simulink model "Casc_Filter_x4"  (Simulink 6.6)
settings: Solver=ode45  StartTime=0.0  StopTime=4100/sampling_freq  RelTol=1e-3
values from neighbouring files (symbols this model uses):
  filter_clk = sampling_freq*clk_mult    (= 144000000)    [Casecade_Taps.m]
  h_g = round(h_g*2^17)/2^17    [Casecade_Taps.m]
  h_k = round(h_k*2^17)/2^17    [Casecade_Taps.m]
  sampling_freq = 48e6    (= 48000000)    [Casecade_Taps.m]
undefined symbols (not defined in the file or in its folder): A, B, Fs, get, PCIN
libraries: xbsIndex_r4 x839, dspsnks4 x5, dspsrcs4 x1, simulink x1
(part 2 of 8)

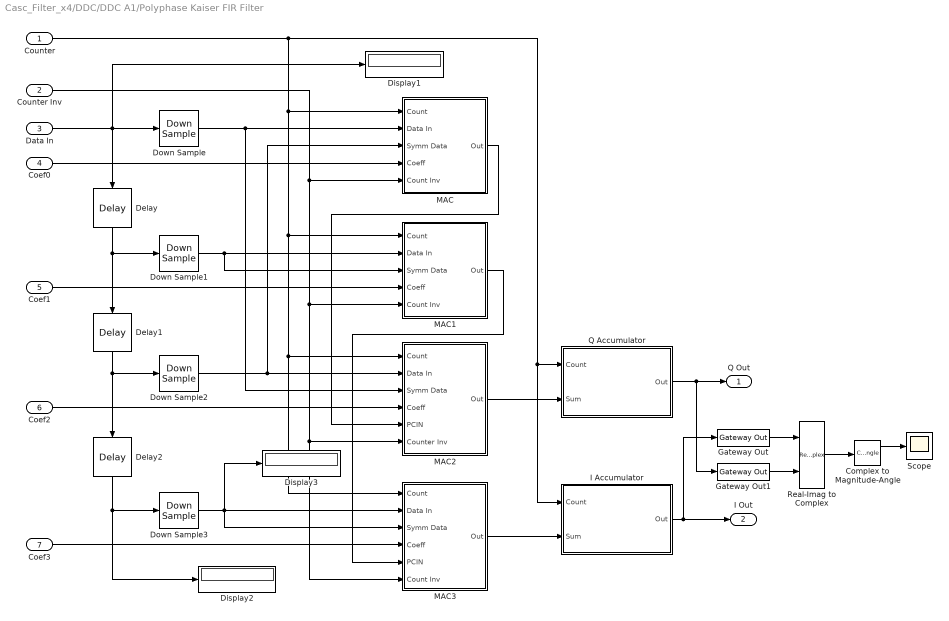
== system Casc_Filter_x4/DDC/DDC A1/Polyphase Kaiser FIR Filter ==
  Counter : Inport
  Counter Inv : Inport  Port=2
  Data In : Inport  Port=3
  Coef0 : Inport  Port=4
  Coef1 : Inport  Port=5
  Coef2 : Inport  Port=6
  Coef3 : Inport  Port=7
  Complex to Magnitude-Angle : ComplexToMagnitudeAngle
  Delay : xbsIndex_r4/Delay  Orientation=down  en=off  latency=1  dbl_ovrd=off  reg_retiming=off  block_type=delay
      settings: infoedit=Hardware notes: A delay line is a chain, each link of which is an SRL16 followed by a flip-flop. If register retiming is enabled, the delay line is a chain of flip-flops.  block_version=8.2
  Delay1 : xbsIndex_r4/Delay  Orientation=down  en=off  latency=1  dbl_ovrd=off  reg_retiming=off  block_type=delay
      settings: infoedit=Hardware notes: A delay line is a chain, each link of which is an SRL16 followed by a flip-flop. If register retiming is enabled, the delay line is a chain of flip-flops.  block_version=8.2
  Delay2 : xbsIndex_r4/Delay  Orientation=down  en=off  latency=1  dbl_ovrd=off  reg_retiming=off  block_type=delay
      settings: infoedit=Hardware notes: A delay line is a chain, each link of which is an SRL16 followed by a flip-flop. If register retiming is enabled, the delay line is a chain of flip-flops.  block_version=8.2
  Display1 : Display
  Display2 : Display
  Display3 : Display
  Down Sample{,1..3} (4 alike) : xbsIndex_r4/Down Sample  sample_ratio=4  sample_phase="Last Value of Frame  (most efficient)"  en=off  latency=1  dbl_ovrd=off  block_type=dsamp
      settings: block_version=8.2
  Gateway Out : xbsIndex_r4/Gateway Out  hdl_port=off  timing_constraint=None  locs_specified=off  LOCs={}  block_type=gatewayout
      settings: infoedit="Gateway out block.  Converts Xilinx fixed point inputs into ouputs of type Simulink integer, double, or fixed point.<P><P>Hardware notes:  In hardware these blocks become top level output ports or are discarded, depending on how they are configured."  block_version=8.2
  Gateway Out1 : xbsIndex_r4/Gateway Out  hdl_port=off  timing_constraint=None  locs_specified=off  LOCs={}  block_type=gatewayout
      settings: infoedit="Gateway out block.  Converts Xilinx fixed point inputs into ouputs of type Simulink integer, double, or fixed point.<P><P>Hardware notes:  In hardware these blocks become top level output ports or are discarded, depending on how they are configured."  block_version=8.2
  I Accumulator : Subsystem
  MAC : Subsystem
  MAC1 : Subsystem
  MAC2 : Subsystem
  MAC3 : Subsystem
  Q Accumulator : Subsystem
  Real-Imag to Complex : RealImagToComplex
  Scope : Scope
  Q Out : Outport
  I Out : Outport  Port=2
  wires:
  Data In/1 -> Down Sample/1, Delay/1, Display1/1
  Delay/1 -> Down Sample1/1, Delay1/1
  Delay1/1 -> Down Sample2/1, Delay2/1
  Delay2/1 -> Down Sample3/1, Display2/1
  Coef0/1 -> MAC/4(Coeff)
  Coef1/1 -> MAC1/4(Coeff)
  I Accumulator/1(Out) -> I Out/1, Gateway Out/1
  Counter/1 -> MAC3/1(Count), MAC2/1(Count), MAC1/1(Count), MAC/1(Count), Q Accumulator/1(Count), I Accumulator/1(Count)
  Coef2/1 -> MAC2/4(Coeff)
  Coef3/1 -> MAC3/4(Coeff)
  Q Accumulator/1(Out) -> Q Out/1, Gateway Out1/1
  Down Sample/1 -> MAC/2(Data In), MAC2/3(Symm Data)
  Down Sample1/1 -> MAC1/3(Symm Data), MAC1/2(Data In)
  Down Sample2/1 -> MAC/3(Symm Data), MAC2/2(Data In)
  Down Sample3/1 -> MAC3/3(Symm Data), MAC3/2(Data In), Display3/1
  MAC/1(Out) -> MAC2/5(PCIN)
  MAC2/1(Out) -> Q Accumulator/2(Sum)
  MAC1/1(Out) -> MAC3/5(PCIN)
  MAC3/1(Out) -> I Accumulator/2(Sum)
  Counter Inv/1 -> MAC/5(Count Inv), MAC1/5(Count Inv), MAC2/6(Counter Inv), MAC3/6(Count Inv)
  Real-Imag to Complex/1 -> Complex to Magnitude-Angle/1
  Complex to Magnitude-Angle/1 -> Scope/1
  Gateway Out/1 -> Real-Imag to Complex/1
  Gateway Out1/1 -> Real-Imag to Complex/2

== system Casc_Filter_x4/DDC/DDC B/Gaussian FIR Filters ==
  Counter : Inport
  Counter Inv : Inport  Port=2
  Q In : Inport  Port=3
  Coef0 : Inport  Port=4
  Coef1 : Inport  Port=5
  Coef2 : Inport  Port=6
  I In : Inport  Port=7
  Gaussian FIR Filter : Subsystem
  Gaussian FIR Filter1 : Subsystem
  I Out : Outport
  Q Out : Outport  Port=2
  wires:
  Counter/1 -> Gaussian FIR Filter/1(Counter), Gaussian FIR Filter1/1(Counter)
  Counter Inv/1 -> Gaussian FIR Filter/2(Counter Inv), Gaussian FIR Filter1/2(Counter Inv)
  Q In/1 -> Gaussian FIR Filter/3(Data In)
  I In/1 -> Gaussian FIR Filter1/3(Data In)
  Gaussian FIR Filter/1(Data Out) -> Q Out/1
  Gaussian FIR Filter1/1(Data Out) -> I Out/1
  Coef0/1 -> Gaussian FIR Filter/4(Coef0), Gaussian FIR Filter1/4(Coef0)
  Coef1/1 -> Gaussian FIR Filter/5(Coef1), Gaussian FIR Filter1/5(Coef1)
  Coef2/1 -> Gaussian FIR Filter/6(Coef2), Gaussian FIR Filter1/6(Coef2)

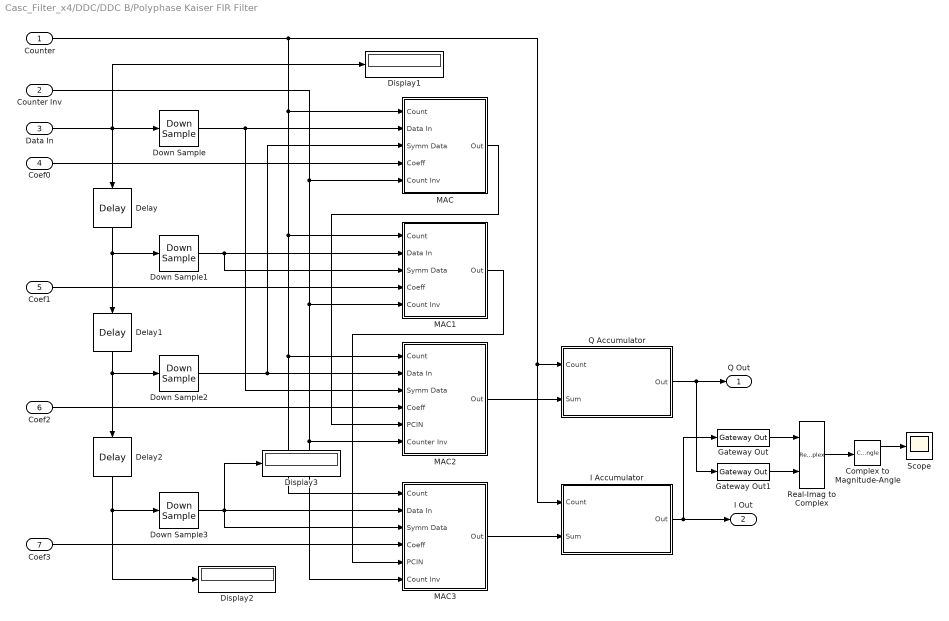
== system Casc_Filter_x4/DDC/DDC B/Polyphase Kaiser FIR Filter ==
  Counter : Inport
  Counter Inv : Inport  Port=2
  Data In : Inport  Port=3
  Coef0 : Inport  Port=4
  Coef1 : Inport  Port=5
  Coef2 : Inport  Port=6
  Coef3 : Inport  Port=7
  Complex to Magnitude-Angle : ComplexToMagnitudeAngle
  Delay : xbsIndex_r4/Delay  Orientation=down  en=off  latency=1  dbl_ovrd=off  reg_retiming=off  block_type=delay
      settings: infoedit=Hardware notes: A delay line is a chain, each link of which is an SRL16 followed by a flip-flop. If register retiming is enabled, the delay line is a chain of flip-flops.  block_version=8.2
  Delay1 : xbsIndex_r4/Delay  Orientation=down  en=off  latency=1  dbl_ovrd=off  reg_retiming=off  block_type=delay
      settings: infoedit=Hardware notes: A delay line is a chain, each link of which is an SRL16 followed by a flip-flop. If register retiming is enabled, the delay line is a chain of flip-flops.  block_version=8.2
  Delay2 : xbsIndex_r4/Delay  Orientation=down  en=off  latency=1  dbl_ovrd=off  reg_retiming=off  block_type=delay
      settings: infoedit=Hardware notes: A delay line is a chain, each link of which is an SRL16 followed by a flip-flop. If register retiming is enabled, the delay line is a chain of flip-flops.  block_version=8.2
  Display1 : Display
  Display2 : Display
  Display3 : Display
  Down Sample{,1..3} (4 alike) : xbsIndex_r4/Down Sample  sample_ratio=4  sample_phase="Last Value of Frame  (most efficient)"  en=off  latency=1  dbl_ovrd=off  block_type=dsamp
      settings: block_version=8.2
  Gateway Out : xbsIndex_r4/Gateway Out  hdl_port=off  timing_constraint=None  locs_specified=off  LOCs={}  block_type=gatewayout
      settings: infoedit="Gateway out block.  Converts Xilinx fixed point inputs into ouputs of type Simulink integer, double, or fixed point.<P><P>Hardware notes:  In hardware these blocks become top level output ports or are discarded, depending on how they are configured."  block_version=8.2
  Gateway Out1 : xbsIndex_r4/Gateway Out  hdl_port=off  timing_constraint=None  locs_specified=off  LOCs={}  block_type=gatewayout
      settings: infoedit="Gateway out block.  Converts Xilinx fixed point inputs into ouputs of type Simulink integer, double, or fixed point.<P><P>Hardware notes:  In hardware these blocks become top level output ports or are discarded, depending on how they are configured."  block_version=8.2
  I Accumulator : Subsystem
  MAC : Subsystem
  MAC1 : Subsystem
  MAC2 : Subsystem
  MAC3 : Subsystem
  Q Accumulator : Subsystem
  Real-Imag to Complex : RealImagToComplex
  Scope : Scope
  Q Out : Outport
  I Out : Outport  Port=2
  wires:
  Data In/1 -> Down Sample/1, Delay/1, Display1/1
  Delay/1 -> Down Sample1/1, Delay1/1
  Delay1/1 -> Down Sample2/1, Delay2/1
  Delay2/1 -> Down Sample3/1, Display2/1
  Coef0/1 -> MAC/4(Coeff)
  Coef1/1 -> MAC1/4(Coeff)
  I Accumulator/1(Out) -> I Out/1, Gateway Out/1
  Counter/1 -> MAC3/1(Count), MAC2/1(Count), MAC1/1(Count), MAC/1(Count), Q Accumulator/1(Count), I Accumulator/1(Count)
  Coef2/1 -> MAC2/4(Coeff)
  Coef3/1 -> MAC3/4(Coeff)
  Q Accumulator/1(Out) -> Q Out/1, Gateway Out1/1
  Down Sample/1 -> MAC/2(Data In), MAC2/3(Symm Data)
  Down Sample1/1 -> MAC1/3(Symm Data), MAC1/2(Data In)
  Down Sample2/1 -> MAC/3(Symm Data), MAC2/2(Data In)
  Down Sample3/1 -> MAC3/3(Symm Data), MAC3/2(Data In), Display3/1
  MAC/1(Out) -> MAC2/5(PCIN)
  MAC2/1(Out) -> Q Accumulator/2(Sum)
  MAC1/1(Out) -> MAC3/5(PCIN)
  MAC3/1(Out) -> I Accumulator/2(Sum)
  Counter Inv/1 -> MAC/5(Count Inv), MAC1/5(Count Inv), MAC2/6(Counter Inv), MAC3/6(Count Inv)
  Real-Imag to Complex/1 -> Complex to Magnitude-Angle/1
  Complex to Magnitude-Angle/1 -> Scope/1
  Gateway Out/1 -> Real-Imag to Complex/1
  Gateway Out1/1 -> Real-Imag to Complex/2

== system Casc_Filter_x4/DDC/DDC C/Gaussian FIR Filters ==
  Counter : Inport
  Counter Inv : Inport  Port=2
  Q In : Inport  Port=3
  Coef0 : Inport  Port=4
  Coef1 : Inport  Port=5
  Coef2 : Inport  Port=6
  I In : Inport  Port=7
  Gaussian FIR Filter : Subsystem
  Gaussian FIR Filter1 : Subsystem
  I Out : Outport
  Q Out : Outport  Port=2
  wires:
  Counter/1 -> Gaussian FIR Filter/1(Counter), Gaussian FIR Filter1/1(Counter)
  Counter Inv/1 -> Gaussian FIR Filter/2(Counter Inv), Gaussian FIR Filter1/2(Counter Inv)
  Q In/1 -> Gaussian FIR Filter/3(Data In)
  I In/1 -> Gaussian FIR Filter1/3(Data In)
  Gaussian FIR Filter/1(Data Out) -> Q Out/1
  Gaussian FIR Filter1/1(Data Out) -> I Out/1
  Coef0/1 -> Gaussian FIR Filter/4(Coef0), Gaussian FIR Filter1/4(Coef0)
  Coef1/1 -> Gaussian FIR Filter/5(Coef1), Gaussian FIR Filter1/5(Coef1)
  Coef2/1 -> Gaussian FIR Filter/6(Coef2), Gaussian FIR Filter1/6(Coef2)

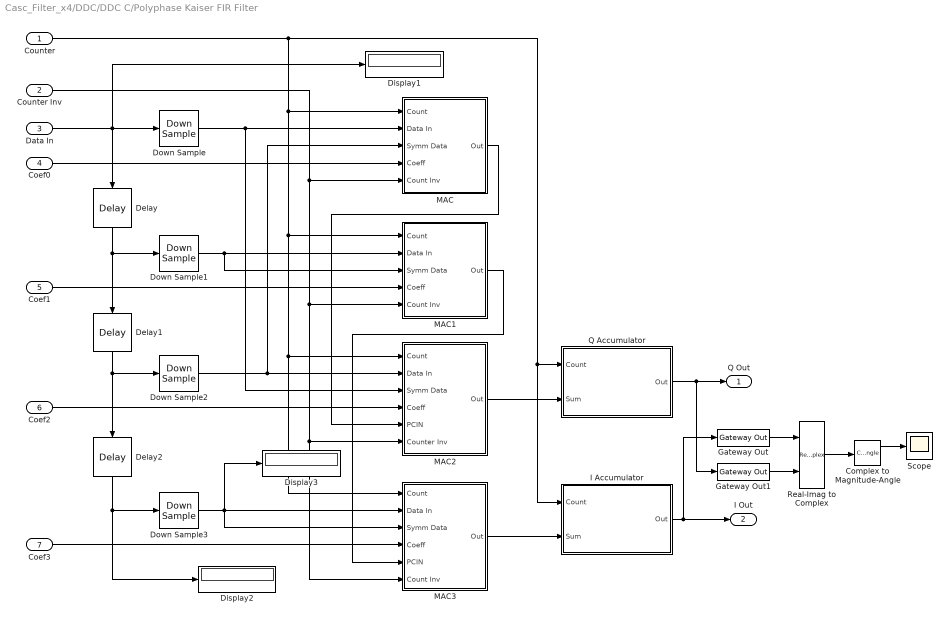
== system Casc_Filter_x4/DDC/DDC C/Polyphase Kaiser FIR Filter ==
  Counter : Inport
  Counter Inv : Inport  Port=2
  Data In : Inport  Port=3
  Coef0 : Inport  Port=4
  Coef1 : Inport  Port=5
  Coef2 : Inport  Port=6
  Coef3 : Inport  Port=7
  Complex to Magnitude-Angle : ComplexToMagnitudeAngle
  Delay : xbsIndex_r4/Delay  Orientation=down  en=off  latency=1  dbl_ovrd=off  reg_retiming=off  block_type=delay
      settings: infoedit=Hardware notes: A delay line is a chain, each link of which is an SRL16 followed by a flip-flop. If register retiming is enabled, the delay line is a chain of flip-flops.  block_version=8.2
  Delay1 : xbsIndex_r4/Delay  Orientation=down  en=off  latency=1  dbl_ovrd=off  reg_retiming=off  block_type=delay
      settings: infoedit=Hardware notes: A delay line is a chain, each link of which is an SRL16 followed by a flip-flop. If register retiming is enabled, the delay line is a chain of flip-flops.  block_version=8.2
  Delay2 : xbsIndex_r4/Delay  Orientation=down  en=off  latency=1  dbl_ovrd=off  reg_retiming=off  block_type=delay
      settings: infoedit=Hardware notes: A delay line is a chain, each link of which is an SRL16 followed by a flip-flop. If register retiming is enabled, the delay line is a chain of flip-flops.  block_version=8.2
  Display1 : Display
  Display2 : Display
  Display3 : Display
  Down Sample{,1..3} (4 alike) : xbsIndex_r4/Down Sample  sample_ratio=4  sample_phase="Last Value of Frame  (most efficient)"  en=off  latency=1  dbl_ovrd=off  block_type=dsamp
      settings: block_version=8.2
  Gateway Out : xbsIndex_r4/Gateway Out  hdl_port=off  timing_constraint=None  locs_specified=off  LOCs={}  block_type=gatewayout
      settings: infoedit="Gateway out block.  Converts Xilinx fixed point inputs into ouputs of type Simulink integer, double, or fixed point.<P><P>Hardware notes:  In hardware these blocks become top level output ports or are discarded, depending on how they are configured."  block_version=8.2
  Gateway Out1 : xbsIndex_r4/Gateway Out  hdl_port=off  timing_constraint=None  locs_specified=off  LOCs={}  block_type=gatewayout
      settings: infoedit="Gateway out block.  Converts Xilinx fixed point inputs into ouputs of type Simulink integer, double, or fixed point.<P><P>Hardware notes:  In hardware these blocks become top level output ports or are discarded, depending on how they are configured."  block_version=8.2
  I Accumulator : Subsystem
  MAC : Subsystem
  MAC1 : Subsystem
  MAC2 : Subsystem
  MAC3 : Subsystem
  Q Accumulator : Subsystem
  Real-Imag to Complex : RealImagToComplex
  Scope : Scope
  Q Out : Outport
  I Out : Outport  Port=2
  wires:
  Data In/1 -> Down Sample/1, Delay/1, Display1/1
  Delay/1 -> Down Sample1/1, Delay1/1
  Delay1/1 -> Down Sample2/1, Delay2/1
  Delay2/1 -> Down Sample3/1, Display2/1
  Coef0/1 -> MAC/4(Coeff)
  Coef1/1 -> MAC1/4(Coeff)
  I Accumulator/1(Out) -> I Out/1, Gateway Out/1
  Counter/1 -> MAC3/1(Count), MAC2/1(Count), MAC1/1(Count), MAC/1(Count), Q Accumulator/1(Count), I Accumulator/1(Count)
  Coef2/1 -> MAC2/4(Coeff)
  Coef3/1 -> MAC3/4(Coeff)
  Q Accumulator/1(Out) -> Q Out/1, Gateway Out1/1
  Down Sample/1 -> MAC/2(Data In), MAC2/3(Symm Data)
  Down Sample1/1 -> MAC1/3(Symm Data), MAC1/2(Data In)
  Down Sample2/1 -> MAC/3(Symm Data), MAC2/2(Data In)
  Down Sample3/1 -> MAC3/3(Symm Data), MAC3/2(Data In), Display3/1
  MAC/1(Out) -> MAC2/5(PCIN)
  MAC2/1(Out) -> Q Accumulator/2(Sum)
  MAC1/1(Out) -> MAC3/5(PCIN)
  MAC3/1(Out) -> I Accumulator/2(Sum)
  Counter Inv/1 -> MAC/5(Count Inv), MAC1/5(Count Inv), MAC2/6(Counter Inv), MAC3/6(Count Inv)
  Real-Imag to Complex/1 -> Complex to Magnitude-Angle/1
  Complex to Magnitude-Angle/1 -> Scope/1
  Gateway Out/1 -> Real-Imag to Complex/1
  Gateway Out1/1 -> Real-Imag to Complex/2

== system Casc_Filter_x4/DDC/Coefficients/Gaus Coef Mem/Select Decoder ==
  Run/Stop : Inport
  Wr/R : Inport  Port=2
  Sel : Inport  Port=3
  BitBasher : xbsIndex_r4/BitBasher  bitexpr=|  display_expr=off  sr_1=1  arith_type1=Unsigned  bin_pt1=0  sr_2=2  arith_type2=Unsigned  bin_pt2=0  sr_3=3  arith_type3=Unsigned  bin_pt3=0  sr_4=4  arith_type4=Unsigned  bin_pt4=0  dbl_ovrd=off  block_type=bitbasher
      | <html><head><meta name="qrichtext" content="1" /></head><body style="font-size:8pt;font-family:MS Shell Dlg">
      | <p>Sel0={Sel[0]}<br />Sel1={Sel[1]}<br /></p>
      | </body></html>
      settings: infoedit="Allows      extraction, concatenation and augmentation of bits"  block_version=VER_STRING_GOES_HERE
  Convert{,1..2,5} (4 alike) : xbsIndex_r4/Convert  arith_type=Boolean  n_bits=16  bin_pt=14  quantization=Truncate  overflow=Wrap  latency=0  dbl_ovrd=off  pipeline=off  block_type=convert
      settings: xl_area=[0 0 0 0 0 0 0]  block_version=VER_STRING_GOES_HERE
  Inverter : xbsIndex_r4/Inverter  en=off  latency=0  dbl_ovrd=off  block_type=inv
      settings: block_version=VER_STRING_GOES_HERE
  Inverter1 : xbsIndex_r4/Inverter  en=off  latency=0  dbl_ovrd=off  block_type=inv
      settings: block_version=VER_STRING_GOES_HERE
  Inverter2 : xbsIndex_r4/Inverter  en=off  latency=0  dbl_ovrd=off  block_type=inv
      settings: block_version=VER_STRING_GOES_HERE
  Logical : xbsIndex_r4/Logical  logical_function=AND  inputs=4  en=off  latency=0  precision=Full  arith_type=Unsigned  n_bits=16  bin_pt=0  align_bp=on  dbl_ovrd=off  block_type=logical
      settings: block_version=VER_STRING_GOES_HERE
  Logical1 : xbsIndex_r4/Logical  logical_function=AND  inputs=4  en=off  latency=0  precision=Full  arith_type=Unsigned  n_bits=16  bin_pt=0  align_bp=on  dbl_ovrd=off  block_type=logical
      settings: block_version=VER_STRING_GOES_HERE
  Logical2 : xbsIndex_r4/Logical  logical_function=AND  inputs=4  en=off  latency=0  precision=Full  arith_type=Unsigned  n_bits=16  bin_pt=0  align_bp=on  dbl_ovrd=off  block_type=logical
      settings: block_version=VER_STRING_GOES_HERE
  Logical3 : xbsIndex_r4/Logical  logical_function=AND  inputs=2  en=off  latency=0  precision=Full  arith_type=Unsigned  n_bits=16  bin_pt=0  align_bp=on  dbl_ovrd=off  block_type=logical
      settings: block_version=VER_STRING_GOES_HERE
  R_En : Outport
  Wr0 : Outport  Port=2
  Wr1 : Outport  Port=3
  Wr2 : Outport  Port=4
  wires:
  BitBasher/1 -> Convert/1
  BitBasher/2 -> Convert1/1
  Sel/1 -> BitBasher/1
  Logical/1 -> Wr0/1
  Logical1/1 -> Wr1/1
  Logical2/1 -> Wr2/1
  Wr/R/1 -> Convert2/1
  Convert/1 -> Inverter/1, Logical1/2
  Convert1/1 -> Inverter1/1, Logical2/3
  Convert2/1 -> Inverter2/1, Logical/1, Logical1/1, Logical2/1
  Inverter/1 -> Logical/2, Logical2/2
  Inverter1/1 -> Logical/3, Logical1/3
  Run/Stop/1 -> Convert5/1
  Convert5/1 -> Logical3/1, Logical/4, Logical1/4, Logical2/4
  Inverter2/1 -> Logical3/2
  Logical3/1 -> R_En/1

== system Casc_Filter_x4/DDC/Coefficients/Poly Coef Mem/Select Decoder ==
  Run/Stop : Inport
  Wr/R : Inport  Port=2
  Sel : Inport  Port=3
  BitBasher : xbsIndex_r4/BitBasher  bitexpr=|  display_expr=off  sr_1=1  arith_type1=Unsigned  bin_pt1=0  sr_2=2  arith_type2=Unsigned  bin_pt2=0  sr_3=3  arith_type3=Unsigned  bin_pt3=0  sr_4=4  arith_type4=Unsigned  bin_pt4=0  dbl_ovrd=off  block_type=bitbasher
      | <html><head><meta name="qrichtext" content="1" /></head><body style="font-size:8pt;font-family:MS Shell Dlg">
      | <p>Sel0={Sel[0]}<br />Sel1={Sel[1]}<br /></p>
      | </body></html>
      settings: infoedit="Allows      extraction, concatenation and augmentation of bits"  block_version=VER_STRING_GOES_HERE
  Convert{,1..2,4} (4 alike) : xbsIndex_r4/Convert  arith_type=Boolean  n_bits=16  bin_pt=14  quantization=Truncate  overflow=Wrap  latency=0  dbl_ovrd=off  pipeline=on  block_type=convert
      settings: xl_area=[0 0 0 0 0 0 0]  block_version=VER_STRING_GOES_HERE
  Inverter : xbsIndex_r4/Inverter  en=off  latency=0  dbl_ovrd=off  block_type=inv
      settings: block_version=VER_STRING_GOES_HERE
  Inverter1 : xbsIndex_r4/Inverter  en=off  latency=0  dbl_ovrd=off  block_type=inv
      settings: block_version=VER_STRING_GOES_HERE
  Inverter2 : xbsIndex_r4/Inverter  en=off  latency=0  dbl_ovrd=off  block_type=inv
      settings: block_version=VER_STRING_GOES_HERE
  Logical{,1..3} (4 alike) : xbsIndex_r4/Logical  logical_function=AND  inputs=4  en=off  latency=0  precision=Full  arith_type=Unsigned  n_bits=16  bin_pt=0  align_bp=on  dbl_ovrd=off  block_type=logical
      settings: block_version=VER_STRING_GOES_HERE
  Logical4 : xbsIndex_r4/Logical  logical_function=AND  inputs=2  en=off  latency=0  precision=Full  arith_type=Unsigned  n_bits=16  bin_pt=0  align_bp=on  dbl_ovrd=off  block_type=logical
      settings: block_version=VER_STRING_GOES_HERE
  R_En : Outport
  Wr0 : Outport  Port=2
  Wr1 : Outport  Port=3
  Wr2 : Outport  Port=4
  Wr3 : Outport  Port=5
  wires:
  BitBasher/1 -> Convert/1
  BitBasher/2 -> Convert1/1
  Sel/1 -> BitBasher/1
  Logical/1 -> Wr0/1
  Logical1/1 -> Wr1/1
  Logical2/1 -> Wr2/1
  Logical3/1 -> Wr3/1
  Wr/R/1 -> Convert2/1
  Convert/1 -> Inverter/1, Logical1/2, Logical3/2
  Convert1/1 -> Inverter1/1, Logical3/3, Logical2/3
  Convert2/1 -> Inverter2/1, Logical/1, Logical1/1, Logical2/1, Logical3/1
  Inverter/1 -> Logical/2, Logical2/2
  Inverter1/1 -> Logical/3, Logical1/3
  Run/Stop/1 -> Convert4/1
  Convert4/1 -> Logical4/1, Logical/4, Logical1/4, Logical2/4, Logical3/4
  Inverter2/1 -> Logical4/2
  Logical4/1 -> R_En/1

== system Casc_Filter_x4/DDC/DDC A/Gaussian FIR Filters/Gaussian FIR Filter ==
  Counter : Inport
  Counter Inv : Inport  Port=2
  Data In : Inport  Port=3
  Coef0 : Inport  Port=4
  Coef1 : Inport  Port=5
  Coef2 : Inport  Port=6
  Gaussian Accumulate : Subsystem
  Gaussian Mult : Subsystem
  Symmetric Data Flow : Subsystem
  Data Out : Outport
  wires:
  Counter/1 -> Gaussian Accumulate/1(Counter), Symmetric Data Flow/2(Counter)
  Gaussian Mult/1(Sum Out) -> Gaussian Accumulate/2(Data In)
  Symmetric Data Flow/1(Data 1) -> Gaussian Mult/1(Data 1)
  Symmetric Data Flow/2(Data 2) -> Gaussian Mult/2(Data 2)
  Data In/1 -> Symmetric Data Flow/1(Data In)
  Gaussian Accumulate/1(Data Out) -> Data Out/1
  Symmetric Data Flow/3(Data 3) -> Gaussian Mult/3(Data 3)
  Coef0/1 -> Gaussian Mult/4(Coeff 1)
  Coef1/1 -> Gaussian Mult/5(Coeff 2)
  Counter Inv/1 -> Symmetric Data Flow/3(Counter Inv)
  Coef2/1 -> Gaussian Mult/6(Coeff 3)

== system Casc_Filter_x4/DDC/DDC A/Gaussian FIR Filters/Gaussian FIR Filter1 ==
  Counter : Inport
  Counter Inv : Inport  Port=2
  Data In : Inport  Port=3
  Coef0 : Inport  Port=4
  Coef1 : Inport  Port=5
  Coef2 : Inport  Port=6
  Gaussian Accumulate : Subsystem
  Gaussian Mult : Subsystem
  Symmetric Data Flow : Subsystem
  Data Out : Outport
  wires:
  Counter/1 -> Gaussian Accumulate/1(Counter), Symmetric Data Flow/2(Counter)
  Gaussian Mult/1(Sum Out) -> Gaussian Accumulate/2(Data In)
  Symmetric Data Flow/1(Data 1) -> Gaussian Mult/1(Data 1)
  Symmetric Data Flow/2(Data 2) -> Gaussian Mult/2(Data 2)
  Data In/1 -> Symmetric Data Flow/1(Data In)
  Gaussian Accumulate/1(Data Out) -> Data Out/1
  Symmetric Data Flow/3(Data 3) -> Gaussian Mult/3(Data 3)
  Coef0/1 -> Gaussian Mult/4(Coeff 1)
  Coef1/1 -> Gaussian Mult/5(Coeff 2)
  Counter Inv/1 -> Symmetric Data Flow/3(Counter Inv)
  Coef2/1 -> Gaussian Mult/6(Coeff 3)

== system Casc_Filter_x4/DDC/DDC A/Polyphase Kaiser FIR Filter/I Accumulator ==
  Count : Inport
  Sum : Inport  Port=2
  Constant : xbsIndex_r4/Constant  arith_type=Signed (2's comp)  const=16383  n_bits=48  bin_pt=0  explicit_period=off  period=1  equ=P=C  opselect=C  inp2=PCIN>>17  opr=+  inp1=P  carry=CIN  dbl_ovrd=off  block_type=constant
      settings: block_version=8.2
  Constant1 : xbsIndex_r4/Constant  arith_type=Unsigned  const=0  n_bits=1  bin_pt=0  explicit_period=off  period=1  equ=P=C  opselect=C  inp2=PCIN>>17  opr=+  inp1=P  carry=CIN  dbl_ovrd=off  block_type=constant
      settings: block_version=8.2
  Constant6 : xbsIndex_r4/Constant  arith_type=Signed (2's comp)  const=0  n_bits=18  bin_pt=0  explicit_period=off  period=1  equ=P=PCIN+(A*B)  opselect=PCIN + A*B  inp2=PCIN>>17  opr=+  inp1=P  carry=CIN  dbl_ovrd=off  block_type=constant
      settings: block_version=8.2
  Constant7 : xbsIndex_r4/Constant  arith_type=Signed (2's comp)  const=0  n_bits=18  bin_pt=0  explicit_period=off  period=1  equ=P=PCIN+(A*B)  opselect=PCIN + A*B  inp2=PCIN>>17  opr=+  inp1=P  carry=CIN  dbl_ovrd=off  block_type=constant
      settings: block_version=8.2
  Constant8 : xbsIndex_r4/Constant  arith_type=DSP48 Instruction  const=1  n_bits=16  bin_pt=14  explicit_period=off  period=1  equ=P=PCIN+(P)  opselect=Custom  inp2=PCIN  opr=+  inp1=P  carry=0  dbl_ovrd=off  block_type=constant
      settings: block_version=8.2
  Constant9 : xbsIndex_r4/Constant  arith_type=DSP48 Instruction  const=1  n_bits=16  bin_pt=14  explicit_period=off  period=1  equ=P=PCIN+(C)  opselect=Custom  inp2=PCIN  opr=+  inp1=C  carry=0  dbl_ovrd=off  block_type=constant
      settings: block_version=8.2
  DSP2 : xbsIndex_r4/DSP48  use_b=Direct from B Port  use_op=on  use_creg=on  use_pcin=on  use_pcout=off  use_bcout=off  rst_all=off  en_all=off  pipeline_a=0  pipeline_b=0  pipeline_c=on  pipeline_p=on  pipeline_mult=off  pipeline_opmode=on  pipeline_sub=off  pipeline_carryin=off  pipeline_carryinsel=off  rst_a=off  rst_b=off  rst_c=off  rst_mult=off  rst_p=off  rst_carry_in=off  rst_ctrl=off  en_a=off  en_b=off  en_c=off  en_mult=off  en_p=off  en_carry_in=off  en_ctrl=off  dbl_ovrd=off  use_synth_model=off  xl_useadderonly=on  block_type=dsp48
      settings: block_version=8.2
  Delay : xbsIndex_r4/Delay  en=off  latency=2  dbl_ovrd=off  reg_retiming=off  block_type=delay
      settings: infoedit=Hardware notes: A delay line is a chain, each link of which is an SRL16 followed by a flip-flop. If register retiming is enabled, the delay line is a chain of flip-flops.  block_version=8.2
  Down Sample1 : xbsIndex_r4/Down Sample  sample_ratio=downsample  sample_phase="Last Value of Frame  (most efficient)"  en=off  latency=1  dbl_ovrd=off  block_type=dsamp
      settings: block_version=8.2
  Mux : xbsIndex_r4/Mux  inputs=2  en=off  latency=1  precision=Full  arith_type=Unsigned  n_bits=16  bin_pt=14  quantization=Truncate  overflow=Wrap  dbl_ovrd=off  block_type=mux
      settings: block_version=8.2
  Register : xbsIndex_r4/Register  init=0  rst=off  en=off  dbl_ovrd=off  block_type=register
      settings: block_version=8.2
  Register1 : xbsIndex_r4/Register  Orientation=down  init=0  rst=off  en=on  dbl_ovrd=off  block_type=register
      settings: block_version=8.2
  Reinterpret : xbsIndex_r4/Reinterpret  force_arith_type=on  arith_type="Signed  (2's comp)"  force_bin_pt=on  bin_pt=17  block_type=reinterpret
      settings: infoedit="Changes signal type without altering the binary representation.   You can changed the signal between signed and unsigned, and relocate the binary point.<P><P>Hardware notes: In hardware this block costs nothing.<P><P>Example:  Suppose the input is 6 bits wide, signed, with 2 fractional bits, and the output is forced to unsigned with 0 fractional bits.  Then an input of -2.0 (1110.00 in binary 2's complement) becomes an output of 56 (111000 in binary)."  block_version=8.2
  Relational : xbsIndex_r4/Relational  mode=a=b  en=off  latency=4  dbl_ovrd=off  block_type=relational
      settings: block_version=8.2
  Slice : xbsIndex_r4/Slice  nbits=16  boolean_output=off  mode=Two Bit Locations  bit1=-15  base1=MSB of Input  bit0=15  base0=LSB of Input  dbl_ovrd=off  block_type=slice
      settings: infoedit="Extracts a given range of bits from each input sample and presents it at the output.  The output type is ordinarily unsigned with binary point at zero, but can be Boolean when the slice is one bit wide.<P><P>Hardware notes: In hardware this block costs nothing."  block_version=8.2
  Out : Outport
  wires:
  Register1/1 -> Down Sample1/1
  Down Sample1/1 -> Slice/1
  Constant1/1 -> Relational/2
  Count/1 -> Relational/1
  Relational/1 -> Mux/1, Delay/1
  Reinterpret/1 -> Register/1
  Constant6/1 -> DSP2/1
  Constant7/1 -> DSP2/2
  DSP2/1 -> Register1/1
  Constant9/1 -> Mux/3
  Constant8/1 -> Mux/2
  Delay/1 -> Register1/2
  Slice/1 -> Reinterpret/1
  Register/1 -> Out/1
  Mux/1 -> DSP2/5
  Sum/1 -> DSP2/4
  Constant/1 -> DSP2/3

== system Casc_Filter_x4/DDC/DDC A/Polyphase Kaiser FIR Filter/MAC ==
  Count : Inport
  Data In : Inport  Port=2
  Symm Data : Inport  Port=3
  Coeff : Inport  Port=4
  Count Inv : Inport  Port=5
  ASR : xbsIndex_r4/Addressable Shift Register  infer_latency=off  depth=12  initVector=[0]  en=off  dbl_ovrd=off  use_behavioral_HDL=off  use_rpm=off  block_type=addrsr
      settings: block_version=8.2
      settings: infoedit=|
      | Delay of  configurable length.  Any element  in the delay
      |     line   can    be   addressed   and   driven    onto   the   output
      |     port.<P><P>Hardware  notes: Implemented  using SRL16s.
      |     If Virtex-4, Virtex-II or Spartan-3 devices are used, multiple SRLC16s are cascaded together.
  ASR1 : xbsIndex_r4/Addressable Shift Register  infer_latency=off  depth=12  initVector=[0]  en=off  dbl_ovrd=off  use_behavioral_HDL=off  use_rpm=off  block_type=addrsr
      settings: block_version=8.2
      settings: infoedit=|
      | Delay of  configurable length.  Any element  in the delay
      |     line   can    be   addressed   and   driven    onto   the   output
      |     port.<P><P>Hardware  notes: Implemented  using SRL16s.
      |     If Virtex-4, Virtex-II or Spartan-3 devices are used, multiple SRLC16s are cascaded together.
  AddSub1 : xbsIndex_r4/AddSub  mode=Subtraction  use_carryin=off  use_carryout=off  en=off  latency=1  precision=User Defined  arith_type="Signed  (2's comp)"  n_bits=18  bin_pt=16  quantization="Round  (unbiased: +/- Inf)"  overflow=Saturate  dbl_ovrd=off  use_behavioral_HDL=off  pipelined=on  use_rpm=on  block_type=addsub
      settings: block_version=8.2
  Constant4 : xbsIndex_r4/Constant  arith_type=DSP48 Instruction  const=5  n_bits=7  bin_pt=0  explicit_period=off  period=1  equ=P=+(A*B)  opselect=A * B  inp2=PCIN>>17  opr=+  inp1=P  carry=CIN  dbl_ovrd=off  block_type=constant
      settings: block_version=VER_STRING_GOES_HERE
  DSP1 : xbsIndex_r4/DSP48  use_b=Direct from B Port  use_op=on  use_creg=off  use_pcin=off  use_pcout=on  use_bcout=off  rst_all=off  en_all=off  pipeline_a=1  pipeline_b=1  pipeline_c=on  pipeline_p=on  pipeline_mult=on  pipeline_opmode=off  pipeline_sub=off  pipeline_carryin=off  pipeline_carryinsel=off  rst_a=off  rst_b=off  rst_c=off  rst_mult=off  rst_p=off  rst_carry_in=off  rst_ctrl=off  en_a=off  en_b=off  en_c=off  en_mult=off  en_p=off  en_carry_in=off  en_ctrl=off  dbl_ovrd=off  use_synth_model=off  xl_useadderonly=off  block_type=dsp48
      settings: block_version=8.2
  Delay : xbsIndex_r4/Delay  en=off  latency=2  dbl_ovrd=off  reg_retiming=off  block_type=delay
      settings: infoedit=Hardware notes: A delay line is a chain, each link of which is an SRL16 followed by a flip-flop. If register retiming is enabled, the delay line is a chain of flip-flops.  block_version=8.2
  Delay3 : xbsIndex_r4/Delay  en=off  latency=12  dbl_ovrd=off  reg_retiming=off  block_type=delay
      settings: infoedit=Hardware notes: A delay line is a chain, each link of which is an SRL16 followed by a flip-flop. If register retiming is enabled, the delay line is a chain of flip-flops.  block_version=8.2
  Register : xbsIndex_r4/Register  init=0  rst=off  en=off  dbl_ovrd=off  block_type=register
      settings: block_version=8.2
  Register1 : xbsIndex_r4/Register  init=0  rst=off  en=off  dbl_ovrd=off  block_type=register
      settings: block_version=8.2
  Reinterpret : xbsIndex_r4/Reinterpret  force_arith_type=on  arith_type="Signed  (2's comp)"  force_bin_pt=on  bin_pt=0  block_type=cast
      settings: infoedit="Changes type of samples without altering their binary representation.<P><P>Hardware notes: In hardware this block costs nothing.<P><P>Example:  Suppose the input is 6 bits wide, signed, with 2 fractional bits, and the output is forced to unsigned with 0 fractional bits.  Then an input of -2.0 (1110.00 in binary 2's complement) becomes an output of 56 (111000 in binary)."  block_version=VER_STRING_GOES_HERE
  Reinterpret1 : xbsIndex_r4/Reinterpret  force_arith_type=on  arith_type="Signed  (2's comp)"  force_bin_pt=on  bin_pt=0  block_type=cast
      settings: infoedit="Changes type of samples without altering their binary representation.<P><P>Hardware notes: In hardware this block costs nothing.<P><P>Example:  Suppose the input is 6 bits wide, signed, with 2 fractional bits, and the output is forced to unsigned with 0 fractional bits.  Then an input of -2.0 (1110.00 in binary 2's complement) becomes an output of 56 (111000 in binary)."  block_version=VER_STRING_GOES_HERE
  Terminator : Terminator
  Out : Outport
  wires:
  Count/1 -> ASR/2
  Data In/1 -> ASR/1
  ASR/1 -> Register/1
  AddSub1/1 -> Reinterpret/1
  Coeff/1 -> Delay/1
  Delay/1 -> Reinterpret1/1
  Register/1 -> AddSub1/2
  Symm Data/1 -> Delay3/1
  Count Inv/1 -> ASR1/2
  Delay3/1 -> ASR1/1
  ASR1/1 -> Register1/1
  Register1/1 -> AddSub1/1
  Reinterpret/1 -> DSP1/1
  Reinterpret1/1 -> DSP1/2
  Constant4/1 -> DSP1/3
  DSP1/2 -> Out/1
  DSP1/1 -> Terminator/1

== system Casc_Filter_x4/DDC/DDC A/Polyphase Kaiser FIR Filter/MAC1 ==
  Count : Inport
  Data In : Inport  Port=2
  Symm Data : Inport  Port=3
  Coeff : Inport  Port=4
  Count Inv : Inport  Port=5
  ASR : xbsIndex_r4/Addressable Shift Register  infer_latency=off  depth=12  initVector=[0]  en=off  dbl_ovrd=off  use_behavioral_HDL=off  use_rpm=off  block_type=addrsr
      settings: block_version=8.2
      settings: infoedit=|
      | Delay of  configurable length.  Any element  in the delay
      |     line   can    be   addressed   and   driven    onto   the   output
      |     port.<P><P>Hardware  notes: Implemented  using SRL16s.
      |     If Virtex-4, Virtex-II or Spartan-3 devices are used, multiple SRLC16s are cascaded together.
  ASR1 : xbsIndex_r4/Addressable Shift Register  infer_latency=off  depth=12  initVector=[0]  en=off  dbl_ovrd=off  use_behavioral_HDL=off  use_rpm=off  block_type=addrsr
      settings: block_version=8.2
      settings: infoedit=|
      | Delay of  configurable length.  Any element  in the delay
      |     line   can    be   addressed   and   driven    onto   the   output
      |     port.<P><P>Hardware  notes: Implemented  using SRL16s.
      |     If Virtex-4, Virtex-II or Spartan-3 devices are used, multiple SRLC16s are cascaded together.
  AddSub1 : xbsIndex_r4/AddSub  mode=Addition  use_carryin=off  use_carryout=off  en=off  latency=1  precision=User Defined  arith_type="Signed  (2's comp)"  n_bits=18  bin_pt=16  quantization="Round  (unbiased: +/- Inf)"  overflow=Saturate  dbl_ovrd=off  use_behavioral_HDL=off  pipelined=on  use_rpm=on  block_type=addsub
      settings: block_version=8.2
  Constant3 : xbsIndex_r4/Constant  arith_type=DSP48 Instruction  const=5  n_bits=7  bin_pt=0  explicit_period=off  period=1  equ=P=+(A*B)  opselect=A * B  inp2=PCIN>>17  opr=+  inp1=P  carry=CIN  dbl_ovrd=off  block_type=constant
      settings: block_version=VER_STRING_GOES_HERE
  DSP48 : xbsIndex_r4/DSP48  use_b=Direct from B Port  use_op=on  use_creg=off  use_pcin=off  use_pcout=on  use_bcout=off  rst_all=off  en_all=off  pipeline_a=1  pipeline_b=1  pipeline_c=on  pipeline_p=on  pipeline_mult=on  pipeline_opmode=off  pipeline_sub=off  pipeline_carryin=off  pipeline_carryinsel=off  rst_a=off  rst_b=off  rst_c=off  rst_mult=off  rst_p=off  rst_carry_in=off  rst_ctrl=off  en_a=off  en_b=off  en_c=off  en_mult=off  en_p=off  en_carry_in=off  en_ctrl=off  dbl_ovrd=off  use_synth_model=off  xl_useadderonly=off  block_type=dsp48
      settings: block_version=8.2
  Delay : xbsIndex_r4/Delay  en=off  latency=2  dbl_ovrd=off  reg_retiming=off  block_type=delay
      settings: infoedit=Hardware notes: A delay line is a chain, each link of which is an SRL16 followed by a flip-flop. If register retiming is enabled, the delay line is a chain of flip-flops.  block_version=8.2
  Delay3 : xbsIndex_r4/Delay  en=off  latency=12  dbl_ovrd=off  reg_retiming=off  block_type=delay
      settings: infoedit=Hardware notes: A delay line is a chain, each link of which is an SRL16 followed by a flip-flop. If register retiming is enabled, the delay line is a chain of flip-flops.  block_version=8.2
  Register : xbsIndex_r4/Register  init=0  rst=off  en=off  dbl_ovrd=off  block_type=register
      settings: block_version=8.2
  Register1 : xbsIndex_r4/Register  init=0  rst=off  en=off  dbl_ovrd=off  block_type=register
      settings: block_version=8.2
  Reinterpret : xbsIndex_r4/Reinterpret  force_arith_type=on  arith_type="Signed  (2's comp)"  force_bin_pt=on  bin_pt=0  block_type=cast
      settings: infoedit="Changes type of samples without altering their binary representation.<P><P>Hardware notes: In hardware this block costs nothing.<P><P>Example:  Suppose the input is 6 bits wide, signed, with 2 fractional bits, and the output is forced to unsigned with 0 fractional bits.  Then an input of -2.0 (1110.00 in binary 2's complement) becomes an output of 56 (111000 in binary)."  block_version=VER_STRING_GOES_HERE
  Reinterpret1 : xbsIndex_r4/Reinterpret  force_arith_type=on  arith_type="Signed  (2's comp)"  force_bin_pt=on  bin_pt=0  block_type=cast
      settings: infoedit="Changes type of samples without altering their binary representation.<P><P>Hardware notes: In hardware this block costs nothing.<P><P>Example:  Suppose the input is 6 bits wide, signed, with 2 fractional bits, and the output is forced to unsigned with 0 fractional bits.  Then an input of -2.0 (1110.00 in binary 2's complement) becomes an output of 56 (111000 in binary)."  block_version=VER_STRING_GOES_HERE
  Terminator : Terminator
  Out : Outport
  wires:
  Count/1 -> ASR/2
  Data In/1 -> ASR/1
  AddSub1/1 -> Reinterpret/1
  Coeff/1 -> Delay/1
  DSP48/2 -> Out/1
  Delay/1 -> Reinterpret1/1
  ASR/1 -> Register/1
  Register/1 -> AddSub1/1
  Symm Data/1 -> Delay3/1
  Count Inv/1 -> ASR1/2
  Delay3/1 -> ASR1/1
  ASR1/1 -> Register1/1
  Register1/1 -> AddSub1/2
  Reinterpret/1 -> DSP48/1
  Reinterpret1/1 -> DSP48/2
  Constant3/1 -> DSP48/3
  DSP48/1 -> Terminator/1

== system Casc_Filter_x4/DDC/DDC A/Polyphase Kaiser FIR Filter/MAC2 ==
  Count : Inport
  Data In : Inport  Port=2
  Symm Data : Inport  Port=3
  Coeff : Inport  Port=4
  PCIN : Inport  Port=5
  Counter Inv : Inport  Port=6
  ASR : xbsIndex_r4/Addressable Shift Register  infer_latency=off  depth=12  initVector=[0]  en=off  dbl_ovrd=off  use_behavioral_HDL=off  use_rpm=off  block_type=addrsr
      settings: block_version=8.2
      settings: infoedit=|
      | Delay of  configurable length.  Any element  in the delay
      |     line   can    be   addressed   and   driven    onto   the   output
      |     port.<P><P>Hardware  notes: Implemented  using SRL16s.
      |     If Virtex-4, Virtex-II or Spartan-3 devices are used, multiple SRLC16s are cascaded together.
  ASR1 : xbsIndex_r4/Addressable Shift Register  infer_latency=off  depth=12  initVector=[0]  en=off  dbl_ovrd=off  use_behavioral_HDL=off  use_rpm=off  block_type=addrsr
      settings: block_version=8.2
      settings: infoedit=|
      | Delay of  configurable length.  Any element  in the delay
      |     line   can    be   addressed   and   driven    onto   the   output
      |     port.<P><P>Hardware  notes: Implemented  using SRL16s.
      |     If Virtex-4, Virtex-II or Spartan-3 devices are used, multiple SRLC16s are cascaded together.
  AddSub1 : xbsIndex_r4/AddSub  mode=Subtraction  use_carryin=off  use_carryout=off  en=off  latency=1  precision=User Defined  arith_type="Signed  (2's comp)"  n_bits=18  bin_pt=16  quantization="Round  (unbiased: +/- Inf)"  overflow=Saturate  dbl_ovrd=off  use_behavioral_HDL=off  pipelined=on  use_rpm=on  block_type=addsub
      settings: block_version=8.2
  Constant3 : xbsIndex_r4/Constant  arith_type=DSP48 Instruction  const=53  n_bits=7  bin_pt=0  explicit_period=off  period=1  equ=P=PCIN+(A*B)  opselect=PCIN + A*B  inp2=PCIN>>17  opr=+  inp1=P  carry=CIN  dbl_ovrd=off  block_type=constant
      settings: block_version=VER_STRING_GOES_HERE
  DSP48 : xbsIndex_r4/DSP48  use_b=Direct from B Port  use_op=on  use_creg=off  use_pcin=on  use_pcout=on  use_bcout=off  rst_all=off  en_all=off  pipeline_a=2  pipeline_b=2  pipeline_c=on  pipeline_p=on  pipeline_mult=on  pipeline_opmode=off  pipeline_sub=off  pipeline_carryin=off  pipeline_carryinsel=off  rst_a=off  rst_b=off  rst_c=off  rst_mult=off  rst_p=off  rst_carry_in=off  rst_ctrl=off  en_a=off  en_b=off  en_c=off  en_mult=off  en_p=off  en_carry_in=off  en_ctrl=off  dbl_ovrd=off  use_synth_model=off  xl_useadderonly=off  block_type=dsp48
      settings: block_version=8.2
  Delay : xbsIndex_r4/Delay  en=off  latency=2  dbl_ovrd=off  reg_retiming=off  block_type=delay
      settings: infoedit=Hardware notes: A delay line is a chain, each link of which is an SRL16 followed by a flip-flop. If register retiming is enabled, the delay line is a chain of flip-flops.  block_version=8.2
  Delay3 : xbsIndex_r4/Delay  en=off  latency=12  dbl_ovrd=off  reg_retiming=off  block_type=delay
      settings: infoedit=Hardware notes: A delay line is a chain, each link of which is an SRL16 followed by a flip-flop. If register retiming is enabled, the delay line is a chain of flip-flops.  block_version=8.2
  Register : xbsIndex_r4/Register  init=0  rst=off  en=off  dbl_ovrd=off  block_type=register
      settings: block_version=8.2
  Register1 : xbsIndex_r4/Register  init=0  rst=off  en=off  dbl_ovrd=off  block_type=register
      settings: block_version=8.2
  Reinterpret : xbsIndex_r4/Reinterpret  force_arith_type=on  arith_type="Signed  (2's comp)"  force_bin_pt=on  bin_pt=0  block_type=cast
      settings: infoedit="Changes type of samples without altering their binary representation.<P><P>Hardware notes: In hardware this block costs nothing.<P><P>Example:  Suppose the input is 6 bits wide, signed, with 2 fractional bits, and the output is forced to unsigned with 0 fractional bits.  Then an input of -2.0 (1110.00 in binary 2's complement) becomes an output of 56 (111000 in binary)."  block_version=VER_STRING_GOES_HERE
  Reinterpret1 : xbsIndex_r4/Reinterpret  force_arith_type=on  arith_type="Signed  (2's comp)"  force_bin_pt=on  bin_pt=0  block_type=cast
      settings: infoedit="Changes type of samples without altering their binary representation.<P><P>Hardware notes: In hardware this block costs nothing.<P><P>Example:  Suppose the input is 6 bits wide, signed, with 2 fractional bits, and the output is forced to unsigned with 0 fractional bits.  Then an input of -2.0 (1110.00 in binary 2's complement) becomes an output of 56 (111000 in binary)."  block_version=VER_STRING_GOES_HERE
  Terminator : Terminator
  Out : Outport
  wires:
  Count/1 -> ASR/2
  Data In/1 -> ASR/1
  AddSub1/1 -> Reinterpret/1
  Coeff/1 -> Delay/1
  Delay/1 -> Reinterpret1/1
  ASR/1 -> Register/1
  PCIN/1 -> DSP48/3
  Register/1 -> AddSub1/1
  Symm Data/1 -> Delay3/1
  Counter Inv/1 -> ASR1/2
  Delay3/1 -> ASR1/1
  ASR1/1 -> Register1/1
  Register1/1 -> AddSub1/2
  Reinterpret/1 -> DSP48/1
  Reinterpret1/1 -> DSP48/2
  Constant3/1 -> DSP48/4
  DSP48/1 -> Terminator/1
  DSP48/2 -> Out/1

== system Casc_Filter_x4/DDC/DDC A/Polyphase Kaiser FIR Filter/MAC3 ==
  Count : Inport
  Data In : Inport  Port=2
  Symm Data : Inport  Port=3
  Coeff : Inport  Port=4
  PCIN : Inport  Port=5
  Count Inv : Inport  Port=6
  ASR : xbsIndex_r4/Addressable Shift Register  infer_latency=off  depth=12  initVector=[0]  en=off  dbl_ovrd=off  use_behavioral_HDL=off  use_rpm=off  block_type=addrsr
      settings: block_version=8.2
      settings: infoedit=|
      | Delay of  configurable length.  Any element  in the delay
      |     line   can    be   addressed   and   driven    onto   the   output
      |     port.<P><P>Hardware  notes: Implemented  using SRL16s.
      |     If Virtex-4, Virtex-II or Spartan-3 devices are used, multiple SRLC16s are cascaded together.
  ASR1 : xbsIndex_r4/Addressable Shift Register  infer_latency=off  depth=12  initVector=[0]  en=off  dbl_ovrd=off  use_behavioral_HDL=off  use_rpm=off  block_type=addrsr
      settings: block_version=8.2
      settings: infoedit=|
      | Delay of  configurable length.  Any element  in the delay
      |     line   can    be   addressed   and   driven    onto   the   output
      |     port.<P><P>Hardware  notes: Implemented  using SRL16s.
      |     If Virtex-4, Virtex-II or Spartan-3 devices are used, multiple SRLC16s are cascaded together.
  AddSub : xbsIndex_r4/AddSub  mode=Addition  use_carryin=off  use_carryout=off  en=off  latency=1  precision=User Defined  arith_type="Signed  (2's comp)"  n_bits=18  bin_pt=16  quantization="Round  (unbiased: +/- Inf)"  overflow=Saturate  dbl_ovrd=off  use_behavioral_HDL=off  pipelined=on  use_rpm=on  block_type=addsub
      settings: block_version=8.2
  Constant : xbsIndex_r4/Constant  arith_type=Unsigned  const=1  n_bits=4  bin_pt=0  explicit_period=off  period=1  equ=P=C  opselect=C  inp2=PCIN>>17  opr=+  inp1=P  carry=CIN  dbl_ovrd=off  block_type=constant
      settings: block_version=8.2
  Constant3 : xbsIndex_r4/Constant  arith_type=DSP48 Instruction  const=53  n_bits=7  bin_pt=0  explicit_period=off  period=1  equ=P=PCIN-(A*B)  opselect=Custom  inp2=PCIN  opr=-  inp1=A*B  carry=0  dbl_ovrd=off  block_type=constant
      settings: block_version=VER_STRING_GOES_HERE
  DSP48 : xbsIndex_r4/DSP48  use_b=Direct from B Port  use_op=on  use_creg=off  use_pcin=on  use_pcout=on  use_bcout=off  rst_all=off  en_all=off  pipeline_a=2  pipeline_b=2  pipeline_c=on  pipeline_p=on  pipeline_mult=on  pipeline_opmode=off  pipeline_sub=off  pipeline_carryin=off  pipeline_carryinsel=off  rst_a=off  rst_b=off  rst_c=off  rst_mult=off  rst_p=off  rst_carry_in=off  rst_ctrl=off  en_a=off  en_b=off  en_c=off  en_mult=off  en_p=off  en_carry_in=off  en_ctrl=off  dbl_ovrd=off  use_synth_model=off  xl_useadderonly=off  block_type=dsp48
      settings: block_version=8.2
  Delay1 : xbsIndex_r4/Delay  en=off  latency=2  dbl_ovrd=off  reg_retiming=off  block_type=delay
      settings: infoedit=Hardware notes: A delay line is a chain, each link of which is an SRL16 followed by a flip-flop. If register retiming is enabled, the delay line is a chain of flip-flops.  block_version=8.2
  Delay3 : xbsIndex_r4/Delay  en=off  latency=11  dbl_ovrd=off  reg_retiming=off  block_type=delay
      settings: infoedit=Hardware notes: A delay line is a chain, each link of which is an SRL16 followed by a flip-flop. If register retiming is enabled, the delay line is a chain of flip-flops.  block_version=8.2
  Display : Display
  Display1 : Display
  Display2 : Display
  Register : xbsIndex_r4/Register  init=0  rst=on  en=off  dbl_ovrd=off  block_type=register
      settings: block_version=8.2
  Register1 : xbsIndex_r4/Register  init=0  rst=off  en=off  dbl_ovrd=off  block_type=register
      settings: block_version=8.2
  Reinterpret : xbsIndex_r4/Reinterpret  force_arith_type=on  arith_type="Signed  (2's comp)"  force_bin_pt=on  bin_pt=0  block_type=cast
      settings: infoedit="Changes type of samples without altering their binary representation.<P><P>Hardware notes: In hardware this block costs nothing.<P><P>Example:  Suppose the input is 6 bits wide, signed, with 2 fractional bits, and the output is forced to unsigned with 0 fractional bits.  Then an input of -2.0 (1110.00 in binary 2's complement) becomes an output of 56 (111000 in binary)."  block_version=VER_STRING_GOES_HERE
  Reinterpret1 : xbsIndex_r4/Reinterpret  force_arith_type=on  arith_type="Signed  (2's comp)"  force_bin_pt=on  bin_pt=0  block_type=cast
      settings: infoedit="Changes type of samples without altering their binary representation.<P><P>Hardware notes: In hardware this block costs nothing.<P><P>Example:  Suppose the input is 6 bits wide, signed, with 2 fractional bits, and the output is forced to unsigned with 0 fractional bits.  Then an input of -2.0 (1110.00 in binary 2's complement) becomes an output of 56 (111000 in binary)."  block_version=VER_STRING_GOES_HERE
  Relational : xbsIndex_r4/Relational  mode=a=b  en=off  latency=1  dbl_ovrd=off  block_type=relational
      settings: block_version=8.2
  Terminator : Terminator
  Out : Outport
  wires:
  Count/1 -> ASR/2
  Data In/1 -> ASR/1
  ASR/1 -> Register1/1, Display2/1
  AddSub/1 -> Reinterpret/1, Display/1
  Coeff/1 -> Delay1/1
  Delay1/1 -> Reinterpret1/1, Display1/1
  PCIN/1 -> DSP48/3
  Register1/1 -> AddSub/1
  Symm Data/1 -> Delay3/1
  Count Inv/1 -> ASR1/2, Relational/1
  Delay3/1 -> ASR1/1
  ASR1/1 -> Register/1
  Constant/1 -> Relational/2
  Relational/1 -> Register/2
  Register/1 -> AddSub/2
  Reinterpret/1 -> DSP48/1
  Reinterpret1/1 -> DSP48/2
  Constant3/1 -> DSP48/4
  DSP48/1 -> Terminator/1
  DSP48/2 -> Out/1
